simulink model "Grua_MC_R2_FFLimitado_06102026"  (R2025b)
settings: Solver=ode23t  StartTime=0.0  StopTime=628  MaxStep=T_s  RelTol=1e-4
InitFcn:
  | addpath(fileparts(get_param('Grua_MC_R2_FFLimitado_06102026','FileName')),'-begin');
  | run(fullfile(fileparts(get_param('Grua_MC_R2_FFLimitado_06102026','FileName')),'definir_buses_variadores.m'));
  | run(fullfile(fileparts(get_param('Grua_MC_R2_FFLimitado_06102026','FileName')),'parametros_ganancias_cascada_29072026.m'));
  | run(fullfile(fileparts(get_param('Grua_MC_R2_FFLimitado_06102026','FileName')),'configurar_modelo_final_hmi.m'));
  | run(fullfile(fileparts(get_param('Grua_MC_R2_FFLimitado_06102026','FileName')),'configurar_parametros_variadores.m'));
  | 
  | 
  | 
  | 
  | 
  | 
  | 
  | Pvis.Ts_viz=.04;Pvis.enable=true;Pvis.keepFigureOnTerminate=true;Pvis.hmi.captureFolder='D:\AyCD\Chat\Proyecto_grua\Prueba_Completa_MC_20261007\corrida_09';Pvis.hmi.fastDiagnostic=false;Pvis.hmi.testDriver=@operador_dos_traslados_v4;Pvis.hmi.renderPeriod=.20;
StopFcn:
  | guardar_prueba_completa;
undefined symbols (not defined in the file): b_cx, b_cy, b_hb, b_hEb, b_heq, b_t, b_tb, b_teq, b_tw, b_wu, g, H_c, HMI, i_h, i_t, J_heq, J_teq, K_cy, K_tw, k_wu, L_h0, l_hi, M_c_profile, M_s, M_t, MC_FF, nLevels0, omega_hmRATED, r_hd, r_td, slotBlock, T_hbMax, T_hEbMax, T_hmMax, T_s, T_s1, T_tbMax, T_tmMax, tau_hm, tau_tm, traj_duration, traj_x_start, traj_x_target, v_hmaxLoaded, v_hmaxUnloaded, x_tmax, x_tmin, Y_c0, Y_t0, Zbase
libraries: simulink x1, aerolibanimutils x1
(part 4 of 5)

== stateflow chart Grua_MC_R2_FFLimitado_06102026/Automata Supervisor ==
  settings: updateMethod=DISCRETE  sampleTime=T_s1  description=Supervisor autocontenido de grua portacontenedores. Ts1=20 ms. El Nivel 0 de seguridad permanece separado y entrega permisos.
  state REFERENCIAS_CARRO_COMUN [parallel]
    entry:
    [xRef,vxRef,axRef,swayTransferVelocity]=referencias_carro_comunes(xRef,vxRef,axRef,modeCode,manualTrolleyRef,xTrolley,enableTrolleyReg,safetyPermitTrolley,swayControlEnable,lastSwayVelocity,TsSupervisor);
    du:
    [xRef,vxRef,axRef,swayTransferVelocity]=referencias_carro_comunes(xRef,vxRef,axRef,modeCode,manualTrolleyRef,xTrolley,enableTrolleyReg,safetyPermitTrolley,swayControlEnable,lastSwayVelocity,TsSupervisor);
    settings: executionOrder=4
  state OPERACION [parallel]
    settings: executionOrder=3
    state APAGADO
      entry:
      modeCode=0; enableTrolleyReg=false; enableHoistReg=false;
      emergencyBrakeHoistOpenCmd=false; swayControlEnable=false;
      xRef=xTrolley; vxRef=0.0; axRef=0.0;
      yRef=yHoist; vyRef=0.0; ayRef=0.0;
    state LISTO
      entry:
      modeCode=2; enableTrolleyReg=true; enableHoistReg=true;
      xRef=xTrolley; vxRef=0.0; axRef=0.0;
      yRef=yHoist; vyRef=0.0; ayRef=0.0;
    state ARRANQUE
      entry:
      modeCode=1; enableTrolleyReg=false; enableHoistReg=false;
      emergencyBrakeHoistOpenCmd=true;
      xRef=xTrolley; vxRef=0.0; axRef=0.0;
      yRef=yHoist; vyRef=0.0; ayRef=0.0;
    state PREPARAR_ESCANEO_LIDAR
      entry:
      swayControlEnable=false;
      modeCode=9; scanActive=true; profileScanComplete=false; profileValid=false;
      scannedObstacleProfile=-20.0*ones(33,1); scanSampleCounts=zeros(33,1);
      scannedObstacleProfile(33)=0.0; scanSampleCounts(33)=1.0;
      autoCycleComplete=false;
      du:
      enableTrolleyReg=safetyPermitTrolley; enableHoistReg=safetyPermitHoist;
      swayControlEnable=false;
      xRef=xTrolley; vxRef=0.0; axRef=0.0;
      yRef=yHoist; vyRef=min(0.5,0.5*max(0.0,39.7-yHoist)); ayRef=0.0;
      exit: scanActive=false;
    state APROXIMACION_FINAL_MANUAL
      entry: modeCode=3;
      du:
      enableTrolleyReg=safetyPermitTrolley; enableHoistReg=safetyPermitHoist;
      swayControlEnable=swayControlSelect;
      [xRef,vxRef,axRef,yRef,vyRef,ayRef]=referenciaDescensoFinal(autoTargetXLatched,yHoist,vHoist,manualHoistRef,TsSupervisor);
    state MANUAL_SUPERVISADO
      entry: modeCode=3;
      du:
      enableTrolleyReg=safetyPermitTrolley; enableHoistReg=safetyPermitHoist;
      swayControlEnable=swayControlSelect;
      [xRef,vxRef,axRef,yRef,vyRef,ayRef]=referenciasManual(xTrolley,vTrolley,yHoist,vHoist,manualTrolleyRef,manualHoistRef,TsSupervisor);
    state IR_EXTREMO_DERECHO
      entry:
      swayControlEnable=false; modeCode=9; scanActive=true;
      du:
      enableTrolleyReg=safetyPermitTrolley; enableHoistReg=safetyPermitHoist;
      swayControlEnable=false;
      xRef=xTrolley; vxRef=calcularVelocidadBarrido(xTrolley,vTrolley,scanSpeed,true); axRef=0.0;
      yRef=yHoist; vyRef=0.0; ayRef=0.0;
      exit: scanActive=false;
    state BUMPLESS_A_MANUAL
      entry: modeCode=7;
      du:
      enableTrolleyReg=safetyPermitTrolley; enableHoistReg=safetyPermitHoist;
      [xRef,vxRef,axRef,yRef,vyRef,ayRef]=referenciasBumpless(xTrolley,vTrolley,yHoist,vHoist,manualTrolleyRef,manualHoistRef,TsSupervisor);
    state BUMPLESS_A_AUTO
      entry: modeCode=8;
      du:
      enableTrolleyReg=safetyPermitTrolley; enableHoistReg=safetyPermitHoist;
      swayControlEnable=swayControlSelect;
      xRef=xTrolley; vxRef=vTrolley; axRef=aTrolley;
      yRef=yHoist; vyRef=vHoist; ayRef=aHoist;
    state BARRIDO_LIDAR_IZQUIERDA
      entry:
      swayControlEnable=false; modeCode=9; scanActive=true;
      du:
      enableTrolleyReg=safetyPermitTrolley; enableHoistReg=safetyPermitHoist;
      swayControlEnable=false;
      [scannedObstacleProfile,scanSampleCounts]=registrarMuestraLidar(scannedObstacleProfile,scanSampleCounts,lidarX,lidarY);
      xRef=xTrolley; vxRef=calcularVelocidadBarrido(xTrolley,vTrolley,scanSpeed,false); axRef=0.0;
      yRef=yHoist; vyRef=0.0; ayRef=0.0;
      exit: scanActive=false;
    state AUTOMATICO
      entry:
      autoTargetXLatched=autoTargetX;
      autoTargetSurfaceLatched=calcularSuperficieObjetivo(safetyEnvelopeProfile,autoTargetXLatched);
      autoApproachTargetY=calcularObjetivoSeguro(safetyEnvelopeProfile,autoTargetXLatched,loadedState,totalSuspendedMass);
      automaticTargetY=autoApproachTargetY;
      state PLANIFICAR
        entry:
        modeCode=4;
        enableTrolleyReg=safetyPermitTrolley;
        enableHoistReg=safetyPermitHoist;
        swayControlEnable=swayControlSelect;
        [xRef,vxRef,axRef,yRef,vyRef,ayRef]=craneTrajectoryGenerator(true,true,xTrolley,vTrolley,aTrolley,yHoist,vHoist,aHoist,autoTargetXLatched,autoApproachTargetY,safetyEnvelopeProfile,totalSuspendedMass,loadedState,spreaderSwayAngle,spreaderSwayRate,TsSupervisor);
        [vyRef,ayRef]=cerrarLazoPosicionIzaje(yRef,vyRef,ayRef,yHoist,vHoist,loadedState,totalSuspendedMass);
      state EJECUTAR
        du:
        enableTrolleyReg=safetyPermitTrolley;
        enableHoistReg=safetyPermitHoist;
        [xRef,vxRef,axRef,yRef,vyRef,ayRef]=craneTrajectoryGenerator(true,false,xTrolley,vTrolley,aTrolley,yHoist,vHoist,aHoist,autoTargetXLatched,autoApproachTargetY,safetyEnvelopeProfile,totalSuspendedMass,loadedState,spreaderSwayAngle,spreaderSwayRate,TsSupervisor);
        % Por encima de la linea de seguridad se prioriza produccion.
        % Al detener el carro se reactiva antisway antes de autorizar el descenso.
        swayControlEnable=swayControlSelect;
        [vyRef,ayRef]=cerrarLazoPosicionIzaje(yRef,vyRef,ayRef,yHoist,vHoist,loadedState,totalSuspendedMass);
        if abs(xTrolley-autoTargetXLatched)<0.08 && abs(yHoist-autoApproachTargetY)<0.15
        autoCycleComplete=true;
        end
      state MANTENER_OBJETIVO
        entry:
        autoCycleComplete=true;
        du:
        swayControlEnable=swayControlSelect;
        xRef=autoTargetXLatched;
        vxRef=0.0;
        axRef=0.0;
        yRef=autoApproachTargetY;
        vyRef=0.0;
        ayRef=0.0;
      (default) -> PLANIFICAR
      PLANIFICAR -> EJECUTAR : [after(1,tick)]
      EJECUTAR -> MANTENER_OBJETIVO : [abs(xTrolley-autoTargetXLatched)<0.08 && abs(yHoist-autoApproachTargetY)<0.15]
    state FINALIZAR_ESCANEO_LIDAR
      entry:
      swayControlEnable=false;
      modeCode=9; scanActive=false; profileScanComplete=true;
      profileValid=verificarCoberturaPerfil(scanSampleCounts);
      profileMaxY=max(scannedObstacleProfile);
      du:
      swayControlEnable=false;
      enableTrolleyReg=safetyPermitTrolley; enableHoistReg=safetyPermitHoist;
      xRef=xTrolley; vxRef=0.0; axRef=0.0;
      yRef=yHoist; vyRef=0.0; ayRef=0.0;
    state PARADA_NORMAL
      entry: modeCode=5; swayControlEnable=false;
      du:
      enableTrolleyReg=safetyPermitTrolley; enableHoistReg=safetyPermitHoist;
      [xRef,vxRef,axRef,yRef,vyRef,ayRef]=referenciasBumpless(xTrolley,vTrolley,yHoist,vHoist,0.0,0.0,TsSupervisor);
    state RETENCION_FALLA
      entry:
      modeCode=6; enableTrolleyReg=false; enableHoistReg=false;
      swayControlEnable=false;
      xRef=xTrolley; vxRef=0.0; axRef=0.0;
      yRef=yHoist; vyRef=0.0; ayRef=0.0;
    (default) -> APAGADO
    ARRANQUE -> PARADA_NORMAL [order 2] : [cmdStop || ~safetyPermitGlobal]
    LISTO -> PARADA_NORMAL [order 3] : [cmdStop || ~safetyPermitGlobal]
    RETENCION_FALLA -> APAGADO : [cmdReset && safetyPermitGlobal && ~trackingFault && ~loadSequenceFault]
    PARADA_NORMAL -> APAGADO : [allStopped]
    APAGADO -> ARRANQUE : [cmdStart && safetyPermitGlobal && configValid]
    ARRANQUE -> LISTO [order 1] : [safetyPermitTrolley && safetyPermitHoist && after(5,tick)]
    FINALIZAR_ESCANEO_LIDAR -> LISTO [order 1] : [allStopped]
    LISTO -> MANUAL_SUPERVISADO [order 1] : [~modeAutoReq && (~scanProfileReq || profileScanComplete)]
    LISTO -> RETENCION_FALLA [order 4] : [trackingFault || loadSequenceFault]
    MANUAL_SUPERVISADO -> PREPARAR_ESCANEO_LIDAR [order 4] : [scanProfileReq && ~profileScanComplete && ~loadedState && allStopped]
    LISTO -> AUTOMATICO [order 2] : [modeAutoReq && cmdAutoStart && profileValid && autoEntryHeightOK && ~overloadDetected]
    LISTO -> PREPARAR_ESCANEO_LIDAR [order 5] : [scanProfileReq && ~profileScanComplete && ~loadedState]
    ARRANQUE -> RETENCION_FALLA [order 3] : [trackingFault || loadSequenceFault]
    BUMPLESS_A_MANUAL -> MANUAL_SUPERVISADO [order 1] : [abs(vTrolley)<0.10 && abs(vHoist)<0.03 && ~autoCycleComplete]
    APROXIMACION_FINAL_MANUAL -> MANUAL_SUPERVISADO [order 1] : [~loadedState]
    PREPARAR_ESCANEO_LIDAR -> PARADA_NORMAL [order 2] : [cmdStop || ~safetyPermitGlobal]
    PREPARAR_ESCANEO_LIDAR -> RETENCION_FALLA [order 3] : [loadSequenceFault]
    MANUAL_SUPERVISADO -> PARADA_NORMAL [order 2] : [cmdStop || ~safetyPermitGlobal]
    PREPARAR_ESCANEO_LIDAR -> IR_EXTREMO_DERECHO [order 1] : [yHoist>=39.65 && abs(vHoist)<0.05]
    BUMPLESS_A_MANUAL -> APROXIMACION_FINAL_MANUAL [order 4] : [abs(vTrolley)<0.10 && abs(vHoist)<0.03 && autoCycleComplete]
    APROXIMACION_FINAL_MANUAL -> PARADA_NORMAL [order 2] : [cmdStop || ~safetyPermitGlobal]
    APROXIMACION_FINAL_MANUAL -> RETENCION_FALLA [order 3] : [trackingFault || loadSequenceFault]
    IR_EXTREMO_DERECHO -> PARADA_NORMAL [order 2] : [cmdStop || ~safetyPermitGlobal]
    IR_EXTREMO_DERECHO -> RETENCION_FALLA [order 3] : [loadSequenceFault]
    IR_EXTREMO_DERECHO -> BARRIDO_LIDAR_IZQUIERDA [order 1] : [normalLimitXMax || (xTrolley>=48.40 && abs(vTrolley)<0.15)]
    MANUAL_SUPERVISADO -> RETENCION_FALLA [order 3] : [trackingFault || loadSequenceFault]
    BUMPLESS_A_MANUAL -> PARADA_NORMAL [order 2] : [cmdStop || ~safetyPermitGlobal]
    MANUAL_SUPERVISADO -> BUMPLESS_A_AUTO [order 1] : [modeAutoReq && cmdAutoStart && ~overloadDetected && profileValid && autoEntryHeightOK && ~operatorOverride && ~autoCycleComplete]
    BUMPLESS_A_AUTO -> PARADA_NORMAL [order 2] : [cmdStop || ~safetyPermitGlobal]
    BUMPLESS_A_AUTO -> RETENCION_FALLA [order 3] : [trackingFault || loadSequenceFault]
    BUMPLESS_A_MANUAL -> RETENCION_FALLA [order 3] : [trackingFault || loadSequenceFault]
    AUTOMATICO -> BUMPLESS_A_MANUAL [order 1] : [operatorOverride || ~modeAutoReq || autoCycleComplete]
    BARRIDO_LIDAR_IZQUIERDA -> PARADA_NORMAL [order 2] : [cmdStop || ~safetyPermitGlobal]
    BARRIDO_LIDAR_IZQUIERDA -> RETENCION_FALLA [order 3] : [loadSequenceFault]
    BARRIDO_LIDAR_IZQUIERDA -> FINALIZAR_ESCANEO_LIDAR [order 1] : [normalLimitXMin || (xTrolley<=-24.50 && abs(vTrolley)<0.15)]
    BUMPLESS_A_AUTO -> AUTOMATICO [order 1] : [after(2,tick)]
    FINALIZAR_ESCANEO_LIDAR -> PARADA_NORMAL [order 2] : [cmdStop || ~safetyPermitGlobal]
    FINALIZAR_ESCANEO_LIDAR -> RETENCION_FALLA [order 3] : [loadSequenceFault]
    AUTOMATICO -> PARADA_NORMAL [order 2] : [cmdStop || ~safetyPermitGlobal]
    AUTOMATICO -> RETENCION_FALLA [order 3] : [trackingFault || loadSequenceFault]
  state FRENOS [parallel]
    settings: executionOrder=5
    state FRENO_IZAJE [parallel]
      settings: executionOrder=2
      state HB_APLICADO
        entry: brakeHoistOpenCmd=false;
      state HB_PRUEBA_TORQUE
        entry: brakeHoistOpenCmd=false;
      state HB_ABIERTO
        entry: brakeHoistOpenCmd=true;
      state HB_APLICANDO
        entry: brakeHoistOpenCmd=true;
        du: brakeHoistOpenCmd=safetyPermitHoist && (abs(vHoist)>=0.03 || abs(yRef-yHoist)>0.05);
      (default) -> HB_APLICADO
      HB_APLICADO -> HB_PRUEBA_TORQUE : [enableHoistReg && (abs(vyRef)>0.01 || abs(yRef-yHoist)>0.05) && safetyPermitHoist]
      HB_APLICANDO -> HB_APLICADO : [abs(vHoist)<0.03 && abs(yRef-yHoist)<=0.05]
      HB_PRUEBA_TORQUE -> HB_APLICADO [order 2] : [after(50,tick)]
      HB_PRUEBA_TORQUE -> HB_ABIERTO [order 1] : [torqueProvenHoist]
      HB_ABIERTO -> HB_APLICANDO : [~enableHoistReg || (modeCode~=4 && abs(vyRef)<=0.01 && abs(yRef-yHoist)<=0.05) || ~safetyPermitHoist]
    state FRENO_CARRO [parallel]
      settings: executionOrder=1
      state TB_APLICADO
        entry: brakeTrolleyOpenCmd=false;
      state TB_PRUEBA_TORQUE
        entry: brakeTrolleyOpenCmd=false;
      state TB_ABIERTO
        entry: brakeTrolleyOpenCmd=true;
      state TB_APLICANDO
        entry: brakeTrolleyOpenCmd=true;
        du: brakeTrolleyOpenCmd=safetyPermitTrolley && (abs(vTrolley)>=0.03 || abs(xRef-xTrolley)>0.03);
      (default) -> TB_APLICADO
      TB_APLICANDO -> TB_APLICADO : [abs(vTrolley)<0.03 && abs(xRef-xTrolley)<=0.03]
      TB_PRUEBA_TORQUE -> TB_APLICADO [order 2] : [after(50,tick)]
      TB_APLICADO -> TB_PRUEBA_TORQUE : [enableTrolleyReg && (abs(vxRef)>0.01 || abs(xRef-xTrolley)>0.03) && safetyPermitTrolley]
      TB_PRUEBA_TORQUE -> TB_ABIERTO [order 1] : [torqueProvenTrolley]
      TB_ABIERTO -> TB_APLICANDO : [~enableTrolleyReg || (abs(vxRef)<=0.01 && abs(xRef-xTrolley)<=0.03) || ~safetyPermitTrolley]
  state INTERLOCKS [parallel]
    du:
    [cmdTwistlockClose,cmdTwistlockOpen,vTrolley,aTrolley,aHoist,normalLimitYMin,normalLimitYMax,trackingFault,torqueProvenTrolley,torqueProvenHoist]=procesarEntradasCrudas(twistlockButton,omegaTrolley,vHoist,yHoist,torqueTrolleyRaw,torqueHoistRaw,xTrolley,xRef,yRef,modeCode,TsSupervisor);
    scanProfileReq=retenerSolicitudHMI(hmiScanRequestRaw,scanActive,profileScanComplete,cmdStop,cmdReset);
    ropeSlack=detectarCuerdaFloja(ropeTension);
    if profileValid && ~scanActive && loadedState~=previousLoadedState
    scannedObstacleProfile=actualizarPerfilPorCarga(scannedObstacleProfile,xTrolley,loadedState);
    end
    previousLoadedState=loadedState;
    safetyEnvelopeProfile=calcularEnvolventeLocal(scannedObstacleProfile);
    autoEntryHeightOK=profileValid && yHoist>=calcularObjetivoSeguro(safetyEnvelopeProfile,xTrolley,loadedState,totalSuspendedMass);
    autoTargetSurfaceLatched=calcularSuperficieObjetivo(safetyEnvelopeProfile,autoTargetXLatched);
    autoApproachTargetY=calcularObjetivoSeguro(safetyEnvelopeProfile,autoTargetXLatched,loadedState,totalSuspendedMass);
    automaticTargetY=autoApproachTargetY;
    if ~modeAutoReq
    autoCycleComplete=false;
    end
    if ~scanProfileReq && ~scanActive
    profileScanComplete=false;
    end
    [loadSupported,operatorOverride,allStopped,atAutoTargetX,atAutoTargetY]=calcularFlagsSupervisor(ropeTension,twistlocksClosedFb,joyTrolley,joyHoist,xTrolley,vTrolley,yHoist,vHoist,autoTargetXLatched,autoApproachTargetY);
    allStopped=allStopped && abs(vxRef)<0.01 && abs(axRef)<0.03 && abs(xRef-xTrolley)<0.08 && abs(swayTransferVelocity)<0.01;
    [manualTrolleyRef,manualHoistRef,vHoistMax]=calcularMandoManual(joyTrolley,joyHoist,loadedState,overloadDetected,totalSuspendedMass,normalLimitXMin,normalLimitXMax,normalLimitYMin,normalLimitYMax);
    profileMaxY=max(scannedObstacleProfile);
    clearanceLineY=max(manualToAutoHeight,min(40.0,profileMaxY+5.18));
    clearanceOK=calcularDespeje(yHoist,clearanceLineY,totalSuspendedMass);
    [alarmCodeCalc,faultCodeCalc]=calcularCodigos(overloadDetected,trackingFault,loadSequenceFault,safetyPermitGlobal);
    watchdogToggle=~watchdogToggle;
    [spreaderStable,spreaderStableCounter]=evaluarEstabilidadSpreader(spreaderSwayAngle,spreaderSwayRate,contact4,cmdTwistlockClose,spreaderStableCounter,TsSupervisor);
    [postLockStable,postLockStableCounter]=evaluarEstabilidadSpreader(spreaderSwayAngle,spreaderSwayRate,contact4,twistlocksClosedFb,postLockStableCounter,TsSupervisor);
    [manualTrolleyRef,manualHoistRef]=aplicarRetencionToma(manualTrolleyRef,manualHoistRef,twistlocksClosedFb,contact4,postLockStable);
    settings: executionOrder=1
  state CARGA_Y_TWISTLOCKS [parallel]
    settings: executionOrder=2
    state VACIO
      entry:
      loadedState=false; overloadDetected=false; pickupModeActive=false;
      twistlockCloseCmd=false; twistlockOpenCmd=false;
      massEstimationEnable=false; massEstimateValid=false;
      estimatedContainerMass=0.0; totalSuspendedMass=15000.0;
    state CERRANDO_TWISTLOCKS
      entry: twistlockCloseCmd=true; twistlockOpenCmd=false;
      exit: twistlockCloseCmd=false;
    state ESPERAR_ESTABILIZACION_SPREADER
      entry:
      twistlockCloseCmd=false; twistlockOpenCmd=false;
      du:
      twistlockCloseCmd=false; twistlockOpenCmd=false;
    state DESPEGUE_SUAVE
      entry:
      loadedState=true; pickupModeActive=true; massEstimationEnable=false;
    state PESAJE
      entry:
      massEstimationEnable=true; pickupModeActive=true;
      massAccum=0.0; massSampleCount=0.0;
      du:
      massAccum=massAccum+Estimar_Masa(ropeTension,twistlocksClosedFb);
      massSampleCount=massSampleCount+1.0;
      estimatedContainerMass=massAccum/max(1.0,massSampleCount);
      totalSuspendedMass=15000.0+estimatedContainerMass;
      exit: massEstimationEnable=false; pickupModeActive=false;
    state CARGADO
      entry:
      loadedState=true; overloadDetected=false; pickupModeActive=false;
      massEstimateValid=true;
    state SOBRECARGA
      entry:
      loadedState=true; overloadDetected=true; pickupModeActive=false;
      massEstimateValid=true;
    state ABRIENDO_TWISTLOCKS
      entry: twistlockOpenCmd=true; twistlockCloseCmd=false;
      exit: twistlockOpenCmd=false;
    state FALLA_TWISTLOCK
      entry: loadSequenceFault=true; twistlockCloseCmd=false; twistlockOpenCmd=false;
      exit: loadSequenceFault=false;
    ESPERAR_ESTABILIZACION_SPREADER -> CERRANDO_TWISTLOCKS [order 1] : [spreaderStable && cmdTwistlockClose && contact4 && safetyPermitHoist]
    (default) -> VACIO
    ESPERAR_ESTABILIZACION_SPREADER -> VACIO [order 2] : [~cmdTwistlockClose || ~contact4]
    VACIO -> ESPERAR_ESTABILIZACION_SPREADER : [cmdTwistlockClose && contact4 && safetyPermitHoist]
    ABRIENDO_TWISTLOCKS -> VACIO [order 1] : [~twistlocksClosedFb]
    FALLA_TWISTLOCK -> VACIO : [cmdReset && ~twistlocksClosedFb]
    CERRANDO_TWISTLOCKS -> FALLA_TWISTLOCK [order 2] : [after(100,tick)]
    CERRANDO_TWISTLOCKS -> DESPEGUE_SUAVE [order 1] : [twistlocksClosedFb]
    ESPERAR_ESTABILIZACION_SPREADER -> FALLA_TWISTLOCK [order 3] : [~safetyPermitHoist || trackingFault]
    DESPEGUE_SUAVE -> ABRIENDO_TWISTLOCKS [order 2] : [cmdTwistlockOpen && contact4]
    DESPEGUE_SUAVE -> PESAJE [order 1] : [~ropeSlack && abs(vHoist)<0.20 && abs(aHoist)<0.05]
    PESAJE -> CARGADO [order 2] : [after(25,tick) && estimatedContainerMass<=50000.0]
    PESAJE -> SOBRECARGA [order 1] : [after(25,tick) && estimatedContainerMass>50000.0]
    SOBRECARGA -> ABRIENDO_TWISTLOCKS : [cmdTwistlockOpen && contact4]
    CARGADO -> ABRIENDO_TWISTLOCKS : [cmdTwistlockOpen && contact4]
    ABRIENDO_TWISTLOCKS -> FALLA_TWISTLOCK [order 2] : [after(100,tick)]
  state DIAGNOSTICO [parallel]
    settings: executionOrder=6
    state DIAG_OK
      du: alarmCode=0.0; faultCode=0.0;
    state ALARMA
      du: alarmCode=alarmCodeCalc; faultCode=0.0;
    state FALLA
      du: faultCode=faultCodeCalc;
    (default) -> DIAG_OK
    DIAG_OK -> ALARMA [order 1] : [overloadDetected]
    FALLA -> DIAG_OK : [cmdReset && ~trackingFault && ~loadSequenceFault && safetyPermitGlobal]
    DIAG_OK -> FALLA [order 2] : [trackingFault || loadSequenceFault || ~safetyPermitGlobal]
    ALARMA -> DIAG_OK [order 2] : [cmdReset && ~overloadDetected]
    ALARMA -> FALLA [order 1] : [trackingFault || loadSequenceFault || ~safetyPermitGlobal]
  data: yReference function_input; velocityPlan function_input; accelerationPlan function_input; yMeasured function_input; velocityMeasured function_input; loaded function_input; velocityCommand function_output; accelerationCommand function_output; totalMassKg function_input; angle function_input; rate function_input; contact function_input; closeRequest function_input; counter function_input; Ts function_input; stable function_output; counter function_output; vxCmd function_input; vyCmd function_input; twistClosed function_input; contact function_input; stable function_input; vxSafe function_output; vySafe function_output; profile function_input; xTarget function_input; surfaceY function_output; buttonRaw function_input; omegaT function_input; vH function_input; yH function_input; torqueTRaw function_input; torqueHRaw function_input; x function_input; xReference function_input; yReference function_input; currentMode function_input; Ts function_input; closeRequest function_output; openRequest function_output; vT function_output; aT function_output; aH function_output; yMin function_output; yMax function_output; trackFault function_output; torqueTProven function_output; torqueHProven function_output; profileIn function_input; countIn function_input; xSensor function_input; ySensor function_input; profileOut function_output; countOut function_output; sampleCounts function_input; valid function_output; x function_input; v function_input; speedRequest function_input; toRight function_input; velocityCommand function_output; profile function_input; envelope function_output; profileIn function_input; x function_input; loadedNow function_input; profileOut function_output; envelope function_input; xTarget function_input; loaded function_input; massKg function_input; yGoal function_output; raw function_input; active function_input; complete function_input; stop function_input; reset function_input; request function_output; ropeTension function_input; ropeSlack function_output; ropeTension function_input; twistlocksClosed function_input; joyX function_input; joyY function_input; x function_input; vx function_input; y function_input; vy function_input; xTarget function_input; yTarget function_input; loadSupported function_output; operatorOverride function_output; allStopped function_output; atTargetX function_output; atTargetY function_output; joyX function_input; joyY function_input; loaded function_input; overload function_input; totalMass function_input; xMinLimit function_input; xMaxLimit function_input; yMinLimit function_input; yMaxLimit function_input; vxManual function_output; vyManual function_output; vyMax function_output; y function_input; clearanceLine function_input; totalMass function_input; clearanceOK function_output; overload function_input; trackingFault function_input; loadFault function_input; safetyGlobal function_input; alarmCode function_output; faultCode function_output; xPlan function_input; vPlan function_input; aPlan function_input; mode function_input; manualVelocity function_input; xMeasured function_input; enabled function_input; permit function_input; E function_input; lastSw function_input; Ts function_input; xr function_output; vr function_output; ar function_output; transfer function_output; enable function_input; reset function_input; xPos function_input; xVel function_input; xAcc function_input; yPos function_input; yVel function_input; yAcc function_input; xTarget function_input; yTarget function_input; obstacleProfile function_input; suspendedMassKg function_input; loaded function_input; swayAngle function_input; swayRate function_input; Ts function_input; xRef function_output; vxRef function_output; axRef function_output; yRef function_output; vyRef function_output; ayRef function_output; x function_input; vx function_input; y function_input; vy function_input; vxCmd function_input; vyCmd function_input; Ts function_input; xRef function_output; vxRef function_output; axRef function_output; yRef function_output; vyRef function_output; ayRef function_output; x function_input; vx function_input; y function_input; vy function_input; vxTarget function_input; vyTarget function_input; Ts function_input; xRef function_output; vxRef function_output; axRef function_output; yRef function_output; vyRef function_output; ayRef function_output; xTarget function_input; y function_input; vy function_input; vyCmd function_input; Ts function_input; xRef function_output; vxRef function_output; axRef function_output; yRef function_output; vyRef function_output; ayRef function_output; F_hw function_input; TLK_Close_FB function_input; masa function_output; cmdStart input boolean size=1; cmdStop input boolean size=1; modeAutoReq input boolean size=1; cmdAutoStart input boolean size=1; cmdReset input boolean size=1; swayControlSelect input boolean size=1; configValid input boolean size=1; twistlockButton input double; contact4 input boolean size=1; twistlocksClosedFb input boolean size=1; normalLimitXMin input boolean size=1; normalLimitXMax input boolean size=1; safetyPermitGlobal input boolean size=1; safetyPermitTrolley input boolean size=1; safetyPermitHoist input boolean size=1; joyTrolley input double size=1; joyHoist input double size=1; xTrolley input double size=1; omegaTrolley input double; yHoist input double size=1; vHoist input double size=1; ropeTension input double size=1; torqueTrolleyRaw input double; torqueHoistRaw input double; autoTargetX input double size=1; enableTrolleyReg output boolean size=1 =0; enableHoistReg output boolean size=1 =0; brakeTrolleyOpenCmd output boolean size=1 =0; brakeHoistOpenCmd output boolean size=1 =0; emergencyBrakeHoistOpenCmd output boolean size=1 =0; twistlockCloseCmd output boolean size=1 =0; twistlockOpenCmd output boolean size=1 =0; swayControlEnable output boolean size=1 =0; loadedState output boolean size=1 =0; overloadDetected output boolean size=1 =0; watchdogToggle output boolean size=1 =0; xRef output double size=1 =0; vxRef output double size=1 =0; axRef output double size=1 =0; yRef output double size=1 =0; vyRef output double size=1 =0; ayRef output double size=1 =0; modeCode output double size=1 =0; alarmCode output double size=1 =0; faultCode output double size=1 =0; ropeSlack local boolean size=1 =0; loadSupported local boolean size=1 =0; operatorOverride local boolean size=1 =0; allStopped local boolean size=1 =0; atAutoTargetX local boolean size=1 =0; atAutoTargetY local boolean size=1 =0; clearanceOK local boolean size=1 =0; loadSequenceFault local boolean size=1 =0; massEstimationEnable local boolean size=1 =0; pickupModeActive local boolean size=1 =0; vHoistMax local double size=1 =0; totalSuspendedMass local double size=1 =15000; alarmCodeCalc local double size=1 =0; faultCodeCalc local double size=1 =0; TsSupervisor local double size=1 =0.02; manualToAutoHeight input double size=1; finalApproachDistance input double size=1; autoApproachTargetY local double size=1 =0; autoCycleComplete local boolean size=1 =0; spreaderSwayAngle input double size=1; spreaderSwayRate input double size=1; hmiScanRequestRaw input boolean; spreaderStable local boolean size=1 =0; spreaderStableCounter local double size=1 =0; postLockStable local boolean size=1 =0; postLockStableCounter local double size=1 =0; cmdTwistlockClose local boolean size=1 =false; cmdTwistlockOpen local boolean size=1 =false; vTrolley local double size=1 =0.0; aTrolley output double size=1 =0.0; aHoist output double size=1 =0.0; trackingFault output boolean size=1 =false; torqueProvenTrolley output boolean size=1 =false; torqueProvenHoist output boolean size=1 =false; autoTargetXLatched local double =0.0; massAccum local double =0.0; massSampleCount local double =0.0; autoTargetSurfaceLatched local double =0.0; lidarX input double size=1; lidarY input double size=1; scanSpeed input double size=1; profileScanComplete output boolean =false; profileValid output boolean =false; scanActive output boolean =false; scannedObstacleProfile output double size=[33 1] =-20.0*ones(33,1); profileMaxY output double =-20.0; automaticTargetY output double =-20.0; scanSampleCounts local double size=[33 1] =zeros(33,1); clearanceLineY output double =0.0; estimatedContainerMass output double size=1 =0; massEstimateValid output boolean size=1 =0; normalLimitYMin output boolean size=1 =false; normalLimitYMax output boolean size=1 =false; manualTrolleyRef output double size=1 =0; manualHoistRef output double size=1 =0; scanProfileReq local boolean size=1; safetyEnvelopeProfile output double size=[33 1] =zeros(33,1); previousLoadedState local boolean size=1 =false; autoEntryHeightOK local boolean size=1 =false; lastSwayVelocity input; swayTransferVelocity output =0
  function [velocityCommand,accelerationCommand] = cerrarLazoPosicionIzaje(yReference,velocityPlan,accelerationPlan,yMeasured,velocityMeasured,loaded,totalMassKg):
    | function [velocityCommand,accelerationCommand] = cerrarLazoPosicionIzaje(yReference,velocityPlan,accelerationPlan,yMeasured,velocityMeasured,loaded,totalMassKg)
    | %#codegen
    | positionGain=0.60;
    | if loaded
    |     massUse=min(65000.0,max(15000.0,totalMassKg));
    |     velocityLimit=min(3.0,max(1.5,97500.0/massUse)); correctionLimit=0.20;
    | else
    |     velocityLimit=3.00; correctionLimit=1.50;
    | end
    | positionError=yReference-yMeasured;
    | if abs(positionError)<=0.05
    |     positionCorrection=0.0;
    | else
    |     effectiveError=positionError-sign(positionError)*0.05;
    |     positionCorrection=min(correctionLimit,max(-correctionLimit,positionGain*effectiveError));
    | end
    | velocityCommand=min(velocityLimit,max(-velocityLimit,velocityPlan+positionCorrection));
    | accelerationCommand=min(0.25,max(-0.25,accelerationPlan+0.05*(velocityCommand-velocityMeasured)));
    | end
  function [stable,counter]=evaluarEstabilidadSpreader(angle,rate,contact,closeRequest,counter,Ts):
    | function [stable,counter]=evaluarEstabilidadSpreader(angle,rate,contact,closeRequest,counter,Ts)
    | %#codegen
    | % Tolerancias: 0.57 grados y 1.15 grados/s durante 1 segundo.
    | % Se limita la oscilacion, no una pequena inclinacion estacionaria.
    | angleLimit=0.010; rateLimit=0.020;
    | requiredSamples=max(1.0,ceil(1.0/max(0.001,Ts)));
    | insideLimits=contact && closeRequest && abs(angle)<=angleLimit && abs(rate)<=rateLimit;
    | if insideLimits
    |     counter=min(requiredSamples,counter+1.0);
    | else
    |     counter=0.0;
    | end
    | stable=counter>=requiredSamples;
    | end
  function [vxSafe,vySafe]=aplicarRetencionToma(vxCmd,vyCmd,twistClosed,contact,stable):
    | function [vxSafe,vySafe]=aplicarRetencionToma(vxCmd,vyCmd,twistClosed,contact,stable)
    | %#codegen
    | holdPickup=twistClosed && contact && ~stable;
    | if holdPickup
    |     vxSafe=0.0; vySafe=0.0;
    | else
    |     vxSafe=vxCmd; vySafe=vyCmd;
    | end
    | end
  function surfaceY = calcularSuperficieObjetivo(profile,xTarget):
    | function surfaceY = calcularSuperficieObjetivo(profile,xTarget)
    | %#codegen
    | xMin=-30.0; slotWidth=2.44; halfContainerWidth=1.22; overlapTolerance=1.0e-6;
    | loadMin=xTarget-halfContainerWidth;
    | loadMax=xTarget+halfContainerWidth;
    | surfaceY=-20.0;
    | for k=1:33
    |     slotMin=xMin+double(k-1)*slotWidth;
    |     slotMax=slotMin+slotWidth;
    |     if slotMax>loadMin+overlapTolerance && slotMin<loadMax-overlapTolerance
    |         surfaceY=max(surfaceY,profile(k));
    |     end
    | end
    | end
  function [closeRequest,openRequest,vT,aT,aH,yMin,yMax,trackFault,torqueTProven,torqueHProven] = procesarEntradasCrudas(buttonRaw,omegaT,vH,yH,torqueTRaw,torqueHRaw,x,xReference,yReference,currentMode,Ts):
    | function [closeRequest,openRequest,vT,aT,aH,yMin,yMax,trackFault,torqueTProven,torqueHProven] = procesarEntradasCrudas(buttonRaw,omegaT,vH,yH,torqueTRaw,torqueHRaw,x,xReference,yReference,currentMode,Ts)
    | %#codegen
    | persistent initialized previousButton toggleState previousVT previousVH trackingTimer
    | if isempty(initialized)
    |     initialized=true; previousButton=false; toggleState=false;
    |     previousVT=0.0; previousVH=0.0;
    |     trackingTimer=0.0;
    | end
    | sampleTime=max(0.001,Ts);
    | button=buttonRaw>=0.5;
    | if button && ~previousButton
    |     toggleState=~toggleState;
    | end
    | previousButton=button; closeRequest=toggleState; openRequest=~toggleState;
    | vT=0.5*omegaT;
    | aT=min(10.0,max(-10.0,(vT-previousVT)/sampleTime));
    | aH=min(10.0,max(-10.0,(vH-previousVH)/sampleTime));
    | previousVT=vT; previousVH=vH;
    | yMin=yH<=-20.0; yMax=yH>=40.0;
    | torqueTProven=abs(torqueTRaw)>=20.0;
    | torqueHProven=abs(torqueHRaw)>=100.0;
    | badX=abs(xReference-x)>2.5;
    | badY=abs(yReference-yH)>max(1.00,2.0*abs(vH)+0.25);
    | automaticMode=currentMode==4.0 || currentMode==8.0;
    | if automaticMode && (badX || badY)
    |     trackingTimer=trackingTimer+sampleTime;
    | else
    |     trackingTimer=0.0;
    | end
    | trackFault=trackingTimer>=3.0;
    | end
  function [profileOut,countOut] = registrarMuestraLidar(profileIn,countIn,xSensor,ySensor):
    | function [profileOut,countOut] = registrarMuestraLidar(profileIn,countIn,xSensor,ySensor)
    | %#codegen
    | profileOut=profileIn; countOut=countIn;
    | xMin=-30.0; slotWidth=2.44;
    | slot=floor((xSensor-xMin)/slotWidth)+1;
    | if slot>=1 && slot<=33
    |     sampleY=min(40.0,max(-20.0,ySensor));
    |     if countOut(slot)<0.5
    |         profileOut(slot)=sampleY;
    |     else
    |         profileOut(slot)=max(profileOut(slot),sampleY);
    |     end
    |     countOut(slot)=countOut(slot)+1.0;
    | end
    | end
  function valid = verificarCoberturaPerfil(sampleCounts):
    | function valid = verificarCoberturaPerfil(sampleCounts)
    | %#codegen
    | valid=true;
    | for k=1:33
    |     if sampleCounts(k)<1.0
    |         valid=false;
    |     end
    | end
    | end
  function velocityCommand = calcularVelocidadBarrido(x,v,speedRequest,toRight):
    | function velocityCommand = calcularVelocidadBarrido(x,v,speedRequest,toRight)
    | speedLimit=min(2.0,max(0.2,abs(speedRequest)));
    | brakingAcceleration=0.15;
    | if toRight
    |     remaining=max(0.0,48.7-x); direction=1.0;
    | else
    |     remaining=max(0.0,x+24.6); direction=-1.0;
    | end
    | velocityCommand=direction*min(speedLimit,sqrt(2.0*brakingAcceleration*remaining));
    | if remaining<=0.0
    |     if toRight && v>0.15
    |         velocityCommand=0.0;
    |     elseif ~toRight && v<-0.15
    |         velocityCommand=0.0;
    |     else
    |         velocityCommand=0.0;
    |     end
    | end
    | end
  function envelope=calcularEnvolventeLocal(profile):
    | function envelope=calcularEnvolventeLocal(profile)
    | %#codegen
    | envelope=zeros(33,1);
    | for k=1:33
    |     left=max(1,k-1); right=min(33,k+1);
    |     envelope(k)=max(profile(left:right));
    | end
    | end
  function profileOut=actualizarPerfilPorCarga(profileIn,x,loadedNow):
    | function profileOut=actualizarPerfilPorCarga(profileIn,x,loadedNow)
    | %#codegen
    | profileOut=profileIn;
    | slot=min(33,max(1,floor((x+30.0)/2.44)+1));
    | if loadedNow
    |     profileOut(slot)=profileOut(slot)-2.59;
    | else
    |     profileOut(slot)=profileOut(slot)+2.59;
    | end
    | end
  function yGoal=calcularObjetivoSeguro(envelope,xTarget,loaded,massKg):
    | function yGoal=calcularObjetivoSeguro(envelope,xTarget,loaded,massKg)
    | %#codegen
    | surface=calcularSuperficieObjetivo(envelope,xTarget);
    | base=surface+2.59+2.59*double(loaded);
    | rope=max(5.0,min(65.0,45.0-base));
    | khw=236.0e6/(2.0*rope+110.0);
    | stretch=max(15000.0,min(65000.0,massKg))*9.80665/(4.0*khw);
    | yGoal=base+stretch;
    | end
  function request=retenerSolicitudHMI(raw,active,complete,stop,reset):
    | function request=retenerSolicitudHMI(raw,active,complete,stop,reset)
    | %#codegen
    | persistent pending previousRaw
    | if isempty(pending), pending=false; previousRaw=false; end
    | if stop || reset || complete
    |  pending=false;
    | elseif raw && ~previousRaw && ~active
    |  pending=true;
    | end
    | previousRaw=raw; request=pending;
    | end
  function ropeSlack = detectarCuerdaFloja(ropeTension):
    | function ropeSlack = detectarCuerdaFloja(ropeTension)
    | %#codegen
    | persistent slackMemory
    | if isempty(slackMemory)
    | slackMemory=true;
    | end
    | if slackMemory
    |     if ropeTension>15000.0
    | slackMemory=false;
    | end
    | else
    |     if ropeTension<12000.0
    | slackMemory=true;
    | end
    | end
    | ropeSlack=slackMemory;
    | end
  function [loadSupported,operatorOverride,allStopped,atTargetX,atTargetY] = calcularFlagsSupervisor(ropeTension,twistlocksClosed,joyX,joyY,x,vx,y,vy,xTarget,yTarget):
    | function [loadSupported,operatorOverride,allStopped,atTargetX,atTargetY] = calcularFlagsSupervisor(ropeTension,twistlocksClosed,joyX,joyY,x,vx,y,vy,xTarget,yTarget)
    | %#codegen
    | loadSupported=twistlocksClosed && ropeTension>30000.0;
    | operatorOverride=abs(joyX)>0.08 || abs(joyY)>0.08;
    | allStopped=abs(vx)<0.03 && abs(vy)<0.03;
    | atTargetX=abs(x-xTarget)<0.03;
    | atTargetY=abs(y-yTarget)<0.10;
    | end
  function [vxManual,vyManual,vyMax] = calcularMandoManual(joyX,joyY,loaded,overload,totalMass,xMinLimit,xMaxLimit,yMinLimit,yMaxLimit):
    | function [vxManual,vyManual,vyMax] = calcularMandoManual(joyX,joyY,loaded,overload,totalMass,xMinLimit,xMaxLimit,yMinLimit,yMaxLimit)
    | %#codegen
    | if loaded
    |     massUse=min(65000.0,max(15000.0,totalMass));
    |     vyMax=min(3.0,max(1.5,97500.0/massUse));
    | else
    |     vyMax=3.0;
    | end
    | if abs(joyX)<=0.05, vxManual=0.0; else, vxManual=4.0*joyX; end
    | if abs(joyY)<=0.05, vyManual=0.0; else, vyManual=vyMax*joyY; end
    | vxManual=min(4.0,max(-4.0,vxManual));
    | vyManual=min(vyMax,max(-vyMax,vyManual));
    | if overload
    |     vxManual=0.0;
    |     vyMax=0.15; % 10%% de la velocidad nominal cargada
    |     vyManual=min(0.0,max(-vyMax,vyManual));
    | end
    | if (xMinLimit && vxManual<0.0) || (xMaxLimit && vxManual>0.0), vxManual=0.0; end
    | if (yMinLimit && vyManual<0.0) || (yMaxLimit && vyManual>0.0), vyManual=0.0; end
    | end
  function clearanceOK = calcularDespeje(y,clearanceLine,totalMass):
    | function clearanceOK = calcularDespeje(y,clearanceLine,totalMass)
    | %#codegen
    | massUse=min(65000.0,max(15000.0,totalMass));
    | lh=max(5.0,min(65.0,45.0-y));
    | khw=236.0e6/(2.0*lh+110.0);
    | cableStretch=massUse*9.80665/(4.0*khw);
    | clearanceOK=(y-cableStretch)>=clearanceLine;
    | end
  function [alarmCode,faultCode] = calcularCodigos(overload,trackingFault,loadFault,safetyGlobal):
    | function [alarmCode,faultCode] = calcularCodigos(overload,trackingFault,loadFault,safetyGlobal)
    | %#codegen
    | alarmCode=0.0;
    | if overload
    |     alarmCode=1.0;
    | end
    | faultCode=0.0;
    | if trackingFault
    |     faultCode=10.0;
    | elseif loadFault
    |     faultCode=11.0;
    | elseif ~safetyGlobal
    |     faultCode=12.0;
    | end
    | end
  function [xr,vr,ar,transfer]=referencias_carro_comunes(xPlan,vPlan,aPlan,mode,manualVelocity,xMeasured,enabled,permit,E,lastSw,Ts):
    | function [xr,vr,ar,transfer]=referencias_carro_comunes(xPlan,vPlan,aPlan,mode,manualVelocity,xMeasured,enabled,permit,E,lastSw,Ts)
    | %#codegen
    | % N1: objetivos distintos; una sola memoria x/v/a, sin predictor de planta.
    | persistent initialized x v a oldE bias
    | if isempty(initialized)
    |  initialized=true;x=xMeasured;v=0.0;a=0.0;oldE=false;bias=0.0;
    | end
    | h=max(0.001,Ts);amax=0.30;jmax=0.50;
    | if ~enabled || ~permit
    |  x=xMeasured;v=0.0;a=0.0;bias=0.0;oldE=false;
    |  xr=x;vr=v;ar=a;transfer=bias;return;
    | end
    | if oldE && ~E
    |  % Transferencia explicita a N1: v_sw en N2 es cero en este mismo cambio.
    |  bias=bias+lastSw;
    | else
    |  bias=bias+min(.25*h,max(-.25*h,-bias));
    | end
    | oldE=E;
    | if mode==4
    |  % El plan AUTO coordinado con izaje aporta su objetivo x/v/a.
    |  goalA=aPlan+1.0*(vPlan-v)+1.0*(xPlan-x);
    | elseif mode==3 || mode==7
    |  goalA=1.0*(manualVelocity-v);
    | elseif mode==9
    |  goalA=1.0*(vPlan-v);
    | else
    |  % READY, transicion a AUTO y parada conservan memoria y frenan a cero.
    |  goalA=-1.0*v;
    | end
    | goalA=min(amax,max(-amax,goalA));
    | aNext=a+min(jmax*h,max(-jmax*h,goalA-a));
    | % Integracion de un segmento de aceleracion lineal (jerk constante).
    | j=(aNext-a)/h;
    | xNext=x+v*h+.5*a*h*h+j*h*h*h/6;
    | vNext=v+.5*(a+aNext)*h;
    | x=xNext;v=vNext;a=aNext;
    | xr=x;vr=v;ar=a;transfer=bias;
    | end
  function [xRef, vxRef, axRef, yRef, vyRef, ayRef] = craneTrajectoryGenerator( ...:
    | function [xRef, vxRef, axRef, yRef, vyRef, ayRef] = craneTrajectoryGenerator( ...
    |     enable, reset, ...
    |     xPos, xVel, xAcc, ...
    |     yPos, yVel, yAcc, ...
    |     xTarget, yTarget, ...
    |     obstacleProfile, ...
    |     suspendedMassKg, loaded, swayAngle, swayRate, Ts)
    | %#codegen
    | % CRANETRAJECTORYGENERATOR
    | % Generador coordinado de referencias de posicion para trolley e izaje.
    | %
    | % Salidas:
    | %   xRef  [m]     : referencia de posicion del trolley.
    | %   vxRef [m/s]   : referencia de velocidad del trolley.
    | %   axRef [m/s^2] : referencia de aceleracion del trolley.
    | %   yRef  [m]     : referencia de posicion del izaje.
    | %   vyRef [m/s]   : referencia de velocidad del izaje.
    | %   ayRef [m/s^2] : referencia de aceleracion del izaje.
    | %
    | % Convencion de coordenadas de la guia:
    | %   x positivo hacia el barco.
    | %   y positivo hacia arriba, con Yt0 = 45 m.
    | %
    | % Uso:
    | %   - Llamar periodicamente con Ts constante.
    | %   - Aplicar reset=true durante al menos una muestra para inicializar.
    | %   - Un flanco ascendente de enable genera una trayectoria nueva.
    | %   - Un cambio de objetivo mientras enable=true provoca replanificacion
    | %     suave desde el estado medido actual.
    | %
    | % Obstaculos:
    | %   obsXMin, obsXMax: intervalo horizontal ocupado por los obstaculos.
    | %   obsYMax: maxima cota superior dentro de ese intervalo.
    | %   Si obsXMax <= obsXMin, se considera que no hay obstaculo intermedio.
    | %
    | % suspendedMassKg es la masa total suspendida:
    | % spreader + headblock + container, entre 15000 y 65000 kg normalmente.
    | 
    | % -------------------------------------------------------------------------
    | % Parametros de la guia y parametros de diseno
    | % -------------------------------------------------------------------------
    | X_MIN = -30.0;
    | X_MAX =  50.0;
    | Y_MIN = -20.0;
    | Y_MAX =  40.0;
    | 
    | VX_MAX = 2.5;       % maxima velocidad de diseno verificable con la planta
    | AX_MAX = 0.3;       % rampa compatible con el seguimiento del accionamiento
    | JX_MAX = 0.5;       % limite de jerk para el traslado productivo
    | 
    | AY_MAX = 0.25;       % conserva tension durante el descenso cargado
    | JY_MAX = 0.10;       % evita transitorios de izaje que aflojen el cable       % Parametro de diseno [m/s^3]
    | % La velocidad cargada se calcula con la masa suspendida.
    | VY_MAX_EMPTY  = 3.00;
    | 
    | YT0 = 45.0;
    | HC = 2.59;
    | WC = 2.44;
    | G = 9.80665;
    | KHWU = 236.0e6;
    | LH0 = 110.0;
    | 
    | VERTICAL_MARGIN = 2.59;       % Parametro de diseno [m]
    | PATH_SWAY_LIMIT = 5.0*pi/180.0;
    | TARGET_CHANGE_TOL = 1.0e-6;
    | MAX_PLAN_TIME = 300.0;  % permite traslados largos a velocidad conservadora
    | 
    | % -------------------------------------------------------------------------
    | % Memoria interna
    | % -------------------------------------------------------------------------
    | persistent initialized prevEnable active validPlan trajectoryTime
    | persistent xCoef xDuration
    | persistent yUpCoef yUpDuration
    | persistent yDownCoef yDownDuration yDownStart
    | persistent savedXTarget savedYTarget
    | 
    | if isempty(initialized)
    |     initialized = true;
    |     prevEnable = false;
    |     active = false;
    |     validPlan = false;
    |     trajectoryTime = 0.0;
    | 
    |     xCoef = zeros(1,6);
    |     xDuration = 0.0;
    |     yUpCoef = zeros(1,6);
    |     yUpDuration = 0.0;
    |     yDownCoef = zeros(1,6);
    |     yDownDuration = 0.0;
    |     yDownStart = 0.0;
    | 
    |     % Inicializacion constante para compatibilidad con MATLAB/PLC Coder.
    |     savedXTarget = 0.0;
    |     savedYTarget = 0.0;
    | end
    | 
    | % Sanitizacion minima de entradas
    | if Ts <= 0.0
    |     TsUse = 0.001;
    | else
    |     TsUse = Ts;
    | end
    | 
    | xGoal = clampValue(xTarget, X_MIN, X_MAX);
    | yGoal = clampValue(yTarget, Y_MIN, Y_MAX);
    | 
    | if reset
    |     prevEnable = false;
    |     active = false;
    |     validPlan = false;
    |     trajectoryTime = 0.0;
    |     savedXTarget = xGoal;
    |     savedYTarget = yGoal;
    |     xRef = clampValue(xPos, X_MIN, X_MAX);
    |     vxRef = clampValue(xVel, -VX_MAX, VX_MAX);
    |     axRef = clampValue(xAcc, -AX_MAX, AX_MAX);
    |     yRef = clampValue(yPos, Y_MIN, Y_MAX);
    |     if loaded
    |         vyLimitReset = hoistSpeedLimit(suspendedMassKg,loaded);
    |     else
    |         vyLimitReset = VY_MAX_EMPTY;
    |     end
    |     vyRef = clampValue(yVel, -vyLimitReset, vyLimitReset);
    |     ayRef = clampValue(yAcc, -AY_MAX, AY_MAX);
    |     return;
    | end
    | 
    | targetChanged = abs(xGoal-savedXTarget) > TARGET_CHANGE_TOL || ...
    |                 abs(yGoal-savedYTarget) > TARGET_CHANGE_TOL;
    | startRequest = enable && (~prevEnable || targetChanged);
    | 
    | if ~enable
    |     active = false;
    |     validPlan = false;
    |     trajectoryTime = 0.0;
    |     prevEnable = false;
    |     xRef = clampValue(xPos, X_MIN, X_MAX);
    |     vxRef = clampValue(xVel, -VX_MAX, VX_MAX);
    |     axRef = clampValue(xAcc, -AX_MAX, AX_MAX);
    |     yRef = clampValue(yPos, Y_MIN, Y_MAX);
    |     if loaded
    |         vyLimitDisabled = hoistSpeedLimit(suspendedMassKg,loaded);
    |     else
    |         vyLimitDisabled = VY_MAX_EMPTY;
    |     end
    |     vyRef = clampValue(yVel, -vyLimitDisabled, vyLimitDisabled);
    |     ayRef = clampValue(yAcc, -AY_MAX, AY_MAX);
    |     return;
    | end
    | 
    | % -------------------------------------------------------------------------
    | % Planificacion en el flanco de enable o ante cambio de objetivo
    | % -------------------------------------------------------------------------
    | if startRequest
    |     savedXTarget = xGoal;
    |     savedYTarget = yGoal;
    |     trajectoryTime = 0.0;
    |     active = true;
    | 
    |     x0 = clampValue(xPos, X_MIN, X_MAX);
    |     y0 = clampValue(yPos, Y_MIN, Y_MAX);
    |     vx0 = clampValue(xVel, -VX_MAX, VX_MAX);
    |     ax0 = clampValue(xAcc, -AX_MAX, AX_MAX);
    |     ay0 = clampValue(yAcc, -AY_MAX, AY_MAX);
    | 
    |     massUse = clampValue(suspendedMassKg, 15000.0, 65000.0);
    |     if loaded
    |         containerHeight = HC;
    |         vyMax = hoistSpeedLimit(suspendedMassKg,loaded);
    |     else
    |         containerHeight = 0.0;
    |         vyMax = VY_MAX_EMPTY;
    |     end
    | 
    |     vy0 = clampValue(yVel, -vyMax, vyMax);
    |     obsXMin=min(x0,xGoal);
    |     obsXMax=max(x0,xGoal);
    |     obsYMax=maximumProfileBetween(obstacleProfile,obsXMin,obsXMax);
    |     hasObstacle=abs(xGoal-x0)>1.0e-6;
    | 
    |     % Altura de izaje necesaria. El estiramiento se obtiene de las
    |     % ecuaciones 4, 5 y 5.a de la guia en equilibrio cuasiestatico.
    |     if hasObstacle
    |         yRequired0 = obsYMax + containerHeight + VERTICAL_MARGIN;
    |         lhEstimate = clampValue(YT0-yRequired0, 5.0, 65.0);
    |         khw = KHWU/(2.0*lhEstimate + LH0);
    |         cableStretch = massUse*G/(4.0*khw);
    |         yRequired = yRequired0 + cableStretch;
    |         yClear = max(max(y0,yGoal),yRequired);
    |         % Se conserva la altura alta de cruce del ciclo original.
    |         yClear = max(yClear,max(obstacleProfile)+5.18);
    |     else
    |         cableStretch = 0.0;
    |         yRequired = max(y0,yGoal);
    |         yClear = yRequired;
    |     end
    | 
    |     % Si el despeje requerido supera el limite mecanico no se inicia.
    |     validPlan = yClear <= Y_MAX + 1.0e-9;
    |     yClear = clampValue(yClear, Y_MIN, Y_MAX);
    | 
    |     % Plan vertical ascendente.
    |     [yUpCoef,yUpDuration,okYUp] = makeMinimumTimeQuintic( ...
    |         y0,vy0,ay0,yClear,0.0,0.0,vyMax,AY_MAX,JY_MAX,TsUse,MAX_PLAN_TIME);
    |     validPlan = validPlan && okYUp;
    | 
    |     % Plan horizontal inicialmente minimo.
    |     [xCoef,xDuration,okX] = makeCruiseProfile( ...
    |         x0,xGoal,VX_MAX,AX_MAX,JX_MAX,MAX_PLAN_TIME);
    |     validPlan = validPlan && okX;
    | 
    |     if validPlan && hasObstacle && xDuration > 0.0
    |         % Se expande horizontalmente la zona por el ancho de la carga y
    |         % por el sway permitido durante la transferencia.
    |         minHoistY = min(min(y0,yGoal),yClear);
    |         maxRopeLength = clampValue(YT0-minHoistY,5.0,65.0);
    |         collisionMargin = 0.5*WC + VERTICAL_MARGIN;
    |         expandedObsMin = obsXMin-collisionMargin;
    |         expandedObsMax = obsXMax+collisionMargin;
    | 
    |         % Si el trolley alcanzaria el obstaculo antes de lograr despeje,
    |         % se aumenta solamente la duracion horizontal. Ambos ejes siguen
    |         % arrancando en t=0, por lo que no hay salto en la referencia.
    |         safe = trajectoryClearsObstacle( ...
    |             xCoef,xDuration,yUpCoef,yUpDuration,yClear, ...
    |             expandedObsMin,expandedObsMax,obstacleProfile, ...
    |             containerHeight,cableStretch,VERTICAL_MARGIN);
    | 
    |         scaleIterations = 0;
    |         while ~safe && xDuration < MAX_PLAN_TIME && scaleIterations < 240
    |             [xCoef,xDuration] = stretchCruiseProfile(xCoef,1.025,MAX_PLAN_TIME);
    | 
    |             safe = trajectoryClearsObstacle( ...
    |                 xCoef,xDuration,yUpCoef,yUpDuration,yClear, ...
    |                 expandedObsMin,expandedObsMax,obstacleProfile, ...
    |                 containerHeight,cableStretch,VERTICAL_MARGIN);
    |             scaleIterations = scaleIterations+1;
    |         end
    | 
    |         validPlan = validPlan && safe;
    | 
    |         % El descenso comienza en cuanto toda la envolvente horizontal de
    |         % la carga ha salido de la zona de obstaculos.
    |         if xGoal >= x0
    |             exitPosition = expandedObsMax;
    |             targetBeyondObstacle = xGoal >= exitPosition;
    |         else
    |             exitPosition = expandedObsMin;
    |             targetBeyondObstacle = xGoal <= exitPosition;
    |         end
    | 
    |         if targetBeyondObstacle
    |             yDownStart = findCrossingTime( ...
    |                 xCoef,xDuration,exitPosition,xGoal>=x0);
    |         else
    |             yDownStart = xDuration;
    |         end
    |     else
    |         yDownStart = xDuration;
    |     end
    | 
    |     % Si no hay obstaculo, se coordina el descenso para terminar junto con
    |     % el trolley, comenzando desde el estado vertical previsto.
    |     if ~hasObstacle
    |         yDownStart = min(xDuration,yUpDuration);
    |     end
    | 
    |     % Estado vertical exacto al comenzar el descenso.
    |     if yDownStart < yUpDuration
    |         [yDown0,vyDown0,ayDown0] = evaluateQuintic( ...
    |             yUpCoef,yDownStart,yUpDuration);
    |     else
    |         yDown0 = yClear;
    |         vyDown0 = 0.0;
    |         ayDown0 = 0.0;
    |     end
    | 
    |     [yDownCoef,yDownDuration,okYDown] = makeMinimumTimeQuintic( ...
    |         yDown0,vyDown0,ayDown0,yGoal,0.0,0.0, ...
    |         vyMax,AY_MAX,JY_MAX,TsUse,MAX_PLAN_TIME);
    |     validPlan = validPlan && okYDown;
    | 
    |     if ~validPlan
    |         active = false;
    |     end
    | end
    | 
    | % -------------------------------------------------------------------------
    | % Evaluacion de la trayectoria
    | % -------------------------------------------------------------------------
    | if active && validPlan
    |     [xRef,vxRef,axRef] = evaluateCruiseProfile( ...
    |         xCoef,trajectoryTime,xDuration);
    | 
    |     if trajectoryTime < yDownStart
    |         [yRef,vyRef,ayRef] = evaluateQuintic( ...
    |             yUpCoef,trajectoryTime,yUpDuration);
    |     else
    |         [yRef,vyRef,ayRef] = evaluateQuintic( ...
    |             yDownCoef,trajectoryTime-yDownStart,yDownDuration);
    |     end
    | 
    |     totalDuration = max(xDuration,yDownStart+yDownDuration);
    |     if trajectoryTime >= totalDuration
    |         xRef = xGoal;
    |         vxRef = 0.0;
    |         axRef = 0.0;
    |         yRef = yGoal;
    |         vyRef = 0.0;
    |         ayRef = 0.0;
    |         % Mantener el plan activo y el reloj saturado para conservar las
    |         % referencias finales hasta reset, disable o replanificacion.
    |         % No volver a las posiciones medidas al terminar la maniobra.
    |         trajectoryTime = totalDuration;
    |     else
    |         finalDescentAtTarget=yDownStart>=xDuration-1.0e-9;
    |         readyForFinalDescent=abs(xPos-xGoal)<=0.08 && abs(xVel)<=0.06 && ...
    |             abs(swayAngle)<=0.0050 && abs(swayRate)<=0.0120;
    |         if finalDescentAtTarget && trajectoryTime>=yDownStart && ~readyForFinalDescent
    |             trajectoryTime=yDownStart;
    |         else
    |             trajectoryTime=trajectoryTime+TsUse;
    |         end
    |     end
    | else
    |     % Comportamiento seguro cuando el plan es inviable: mantener la
    |     % posicion medida y no generar movimiento automatico.
    |     xRef = clampValue(xPos,X_MIN,X_MAX);
    |     vxRef = clampValue(xVel,-VX_MAX,VX_MAX);
    |     axRef = clampValue(xAcc,-AX_MAX,AX_MAX);
    |     yRef = clampValue(yPos,Y_MIN,Y_MAX);
    |     if loaded
    |         vyLimitInvalid = hoistSpeedLimit(suspendedMassKg,loaded);
    |     else
    |         vyLimitInvalid = VY_MAX_EMPTY;
    |     end
    |     vyRef = clampValue(yVel,-vyLimitInvalid,vyLimitInvalid);
    |     ayRef = clampValue(yAcc,-AY_MAX,AY_MAX);
    | end
    | 
    | xRef = clampValue(xRef,X_MIN,X_MAX);
    | vxRef = clampValue(vxRef,-VX_MAX,VX_MAX);
    | axRef = clampValue(axRef,-AX_MAX,AX_MAX);
    | yRef = clampValue(yRef,Y_MIN,Y_MAX);
    | if loaded
    |     vyLimitOutput = hoistSpeedLimit(suspendedMassKg,loaded);
    | else
    |     vyLimitOutput = VY_MAX_EMPTY;
    | end
    | vyRef = clampValue(vyRef,-vyLimitOutput,vyLimitOutput);
    | ayRef = clampValue(ayRef,-AY_MAX,AY_MAX);
    | prevEnable = enable;
    | end
    | 
    | % =========================================================================
    | % Funciones auxiliares compatibles con generacion de codigo
    | % =========================================================================
    | 
    | function maximumY = maximumProfileBetween(profile,xStart,xEnd)
    | xMin=-30.0; slotWidth=2.44; halfWidth=1.22;
    | pathMin=min(xStart,xEnd)-halfWidth;
    | pathMax=max(xStart,xEnd)+halfWidth;
    | maximumY=-20.0;
    | for k=1:33
    |     slotX=xMin+double(k-1)*slotWidth;
    |     if slotX+halfWidth>=pathMin && slotX-halfWidth<=pathMax
    |         maximumY=max(maximumY,profile(k));
    |     end
    | end
    | end
    | 
    | function value = clampValue(value,lowerLimit,upperLimit)
    | value = min(upperLimit,max(lowerLimit,value));
    | end
    | 
    | function [profile,duration,ok] = makeCruiseProfile( ...
    |     xStart,xGoal,vMax,aMax,jMax,maxTime)
    | distance=abs(xGoal-xStart);
    | if distance<1.0e-10
    |     profile=[xGoal,xGoal,0.0,0.0,0.0,0.0];
    |     duration=0.0; ok=true; return;
    | end
    | direction=sign(xGoal-xStart);
    | rampA=pi*vMax/(2.0*max(aMax,1.0e-6));
    | rampJ=pi*sqrt(vMax/(2.0*max(jMax,1.0e-6)));
    | rampDuration=max(0.25,max(rampA,rampJ));
    | if distance>=vMax*rampDuration
    |     cruiseVelocity=vMax;
    |     cruiseDuration=distance/cruiseVelocity-rampDuration;
    | else
    |     cruiseVelocity=distance/rampDuration;
    |     cruiseDuration=0.0;
    | end
    | duration=2.0*rampDuration+cruiseDuration;
    | profile=[xStart,xGoal,direction,cruiseVelocity,rampDuration,cruiseDuration];
    | ok=duration<=maxTime;
    | end
    | 
    | function [profile,duration] = stretchCruiseProfile(profile,scale,maxTime)
    | oldDuration=2.0*profile(5)+profile(6);
    | newDuration=min(maxTime,scale*oldDuration);
    | actualScale=max(1.0,newDuration/max(oldDuration,1.0e-9));
    | profile(4)=profile(4)/actualScale;
    | profile(5)=profile(5)*actualScale;
    | profile(6)=profile(6)*actualScale;
    | duration=2.0*profile(5)+profile(6);
    | end
    | 
    | function [position,velocity,acceleration] = evaluateCruiseProfile(profile,time,duration)
    | xStart=profile(1); xGoal=profile(2); direction=profile(3);
    | vCruise=profile(4); rampDuration=profile(5);
    | cruiseDuration=profile(6);
    | if duration<=0.0 || direction==0.0
    |     position=xGoal; velocity=0.0; acceleration=0.0; return;
    | end
    | t=min(duration,max(0.0,time));
    | if t<rampDuration
    |     angle=pi*t/rampDuration;
    |     travelled=0.5*vCruise*(t-rampDuration*sin(angle)/pi);
    |     speed=0.5*vCruise*(1.0-cos(angle));
    |     accel=0.5*vCruise*pi*sin(angle)/rampDuration;
    | elseif t<rampDuration+cruiseDuration
    |     travelled=0.5*vCruise*rampDuration+vCruise*(t-rampDuration);
    |     speed=vCruise; accel=0.0;
    | elseif t<duration
    |     tau=t-rampDuration-cruiseDuration;
    |     angle=pi*tau/rampDuration;
    |     travelled=0.5*vCruise*rampDuration+vCruise*cruiseDuration+...
    |         0.5*vCruise*(tau+rampDuration*sin(angle)/pi);
    |     speed=0.5*vCruise*(1.0+cos(angle));
    |     accel=-0.5*vCruise*pi*sin(angle)/rampDuration;
    | else
    |     position=xGoal; velocity=0.0; acceleration=0.0; return;
    | end
    | position=xStart+direction*travelled;
    | velocity=direction*speed; acceleration=direction*accel;
    | end
    | 
    | function [coef,duration,ok] = makeMinimumTimeQuintic( ...
    |     p0,v0,a0,pf,vf,af,vMax,aMax,jMax,Ts,maxTime)
    | 
    | if abs(pf-p0) < 1.0e-10 && abs(v0-vf) < 1.0e-8 && ...
    |         abs(a0-af) < 1.0e-7
    |     coef = [pf,0.0,0.0,0.0,0.0,0.0];
    |     duration = 0.0;
    |     ok = true;
    |     return;
    | end
    | 
    | durationHigh = max(10.0*Ts,0.05);
    | coef = quinticCoefficients(p0,v0,a0,pf,vf,af,durationHigh);
    | 
    | while ~profileWithinLimits(coef,durationHigh,vMax,aMax,jMax) && ...
    |         durationHigh < maxTime
    |     durationHigh = min(maxTime,2.0*durationHigh);
    |     coef = quinticCoefficients(p0,v0,a0,pf,vf,af,durationHigh);
    | end
    | 
    | ok = profileWithinLimits(coef,durationHigh,vMax,aMax,jMax);
    | if ~ok
    |     duration = durationHigh;
    |     return;
    | end
    | 
    | durationLow = max(Ts,0.001);
    | for iteration = 1:48
    |     durationMid = 0.5*(durationLow+durationHigh);
    |     coefMid = quinticCoefficients(p0,v0,a0,pf,vf,af,durationMid);
    |     if profileWithinLimits(coefMid,durationMid,vMax,aMax,jMax)
    |         durationHigh = durationMid;
    |         coef = coefMid;
    |     else
    |         durationLow = durationMid;
    |     end
    | end
    | 
    | duration = durationHigh;
    | end
    | 
    | function coef = quinticCoefficients(p0,v0,a0,pf,vf,af,T)
    | if T <= 0.0
    |     coef = [pf,0.0,0.0,0.0,0.0,0.0];
    |     return;
    | end
    | 
    | T2 = T*T;
    | T3 = T2*T;
    | T4 = T3*T;
    | T5 = T4*T;
    | 
    | c0 = p0;
    | c1 = v0;
    | c2 = 0.5*a0;
    | c3 = (20.0*(pf-p0) - (8.0*vf+12.0*v0)*T ...
    |       - (3.0*a0-af)*T2)/(2.0*T3);
    | c4 = (30.0*(p0-pf) + (14.0*vf+16.0*v0)*T ...
    |       + (3.0*a0-2.0*af)*T2)/(2.0*T4);
    | c5 = (12.0*(pf-p0) - (6.0*vf+6.0*v0)*T ...
    |       - (a0-af)*T2)/(2.0*T5);
    | 
    | coef = [c0,c1,c2,c3,c4,c5];
    | end
    | 
    | function [position,velocity,acceleration] = evaluateQuintic(coef,time,duration)
    | if duration <= 0.0
    |     position = coef(1);
    |     velocity = 0.0;
    |     acceleration = 0.0;
    |     return;
    | end
    | 
    | t = clampValue(time,0.0,duration);
    | c0 = coef(1);
    | c1 = coef(2);
    | c2 = coef(3);
    | c3 = coef(4);
    | c4 = coef(5);
    | c5 = coef(6);
    | 
    | position = c0+t*(c1+t*(c2+t*(c3+t*(c4+t*c5))));
    | velocity = c1+t*(2.0*c2+t*(3.0*c3+t*(4.0*c4+t*5.0*c5)));
    | acceleration = 2.0*c2+t*(6.0*c3+t*(12.0*c4+t*20.0*c5));
    | end
    | 
    | function jerk = evaluateJerk(coef,time,duration)
    | if duration <= 0.0
    |     jerk = 0.0;
    |     return;
    | end
    | t = clampValue(time,0.0,duration);
    | jerk = 6.0*coef(4)+t*(24.0*coef(5)+t*60.0*coef(6));
    | end
    | 
    | function ok = profileWithinLimits(coef,duration,vMax,aMax,jMax)
    | if duration <= 0.0
    |     ok = true;
    |     return;
    | end
    | 
    | ok = true;
    | for sample = 0:240
    |     t = duration*double(sample)/240.0;
    |     [~,velocity,acceleration] = evaluateQuintic(coef,t,duration);
    |     jerk = evaluateJerk(coef,t,duration);
    |     if abs(velocity) > vMax*(1.0+1.0e-8) || ...
    |        abs(acceleration) > aMax*(1.0+1.0e-8) || ...
    |        abs(jerk) > jMax*(1.0+1.0e-8)
    |         ok = false;
    |         return;
    |     end
    | end
    | end
    | 
    | function safe = trajectoryClearsObstacle( ...
    |     xCoef,xDuration,yCoef,yDuration,yHold, ...
    |     obstacleMin,obstacleMax,obstacleProfile, ...
    |     containerHeight,cableStretch,verticalMargin)
    | 
    | safe = true;
    | for sample = 0:400
    |     t = xDuration*double(sample)/400.0;
    |     [x,~,~] = evaluateCruiseProfile(xCoef,t,xDuration);
    | 
    |     if x >= obstacleMin && x <= obstacleMax && abs(x-xCoef(1))>0.02 && abs(x-xCoef(1))>0.02 && abs(x-xCoef(1))>0.02 && abs(x-xCoef(1))>0.02 && abs(x-xCoef(1))>0.02 && abs(x-xCoef(1))>0.02 && abs(x-xCoef(1))>0.02
    |         if t < yDuration
    |             [y,~,~] = evaluateQuintic(yCoef,t,yDuration);
    |         else
    |             y = yHold;
    |         end
    | 
    |         obstacleHeight=maximumProfileBetween(obstacleProfile,x,x);
    |         bottomHeight = y-cableStretch-containerHeight;
    |         if bottomHeight < obstacleHeight+verticalMargin-1.0e-8
    |             safe = false;
    |             return;
    |         end
    |     end
    | end
    | end
    | 
    | function crossingTime = findCrossingTime(coef,duration,position,positiveDirection)
    | crossingTime = duration;
    | if duration <= 0.0
    |     return;
    | end
    | 
    | previousTime = 0.0;
    | [previousPosition,~,~] = evaluateCruiseProfile(coef,0.0,duration);
    | 
    | for sample = 1:400
    |     currentTime = duration*double(sample)/400.0;
    |     [currentPosition,~,~] = evaluateCruiseProfile( ...
    |         coef,currentTime,duration);
    | 
    |     if positiveDirection
    |         crossed = previousPosition < position && currentPosition >= position;
    |     else
    |         crossed = previousPosition > position && currentPosition <= position;
    |     end
    | 
    |     if crossed
    |         low = previousTime;
    |         high = currentTime;
    |         for iteration = 1:32
    |             middle = 0.5*(low+high);
    |             [middlePosition,~,~] = evaluateCruiseProfile(coef,middle,duration);
    |             if positiveDirection
    |                 if middlePosition >= position
    |                     high = middle;
    |                 else
    |                     low = middle;
    |                 end
    |             else
    |                 if middlePosition <= position
    |                     high = middle;
    |                 else
    |                     low = middle;
    |                 end
    |             end
    |         end
    |         crossingTime = high;
    |         return;
    |     end
    | 
    |     previousTime = currentTime;
    |     previousPosition = currentPosition;
    | end
    | end
    | 
    | 
    | function vMax = hoistSpeedLimit(totalMassKg,loaded)
    | if loaded
    |     massUse=clampValue(totalMassKg,15000.0,65000.0);
    |     vMax=min(3.0,max(1.5,97500.0/massUse));
    | else
    |     vMax=3.0;
    | end
    | end
  function [xRef,vxRef,axRef,yRef,vyRef,ayRef] = referenciasManual(x,vx,y,vy,vxCmd,vyCmd,Ts):
    | function [xRef,vxRef,axRef,yRef,vyRef,ayRef] = referenciasManual(x,vx,y,vy,vxCmd,vyCmd,Ts)
    | %#codegen
    | persistent previousVxRef previousVyRef
    | if isempty(previousVxRef)
    |     previousVxRef=0.0; previousVyRef=0.0;
    | end
    | TsUse=max(0.001,Ts);
    | vxTarget=min(4.0,max(-4.0,vxCmd));
    | vyTarget=min(3.0,max(-3.0,vyCmd));
    | deltaVx=min(0.8*TsUse,max(-0.8*TsUse,vxTarget-previousVxRef));
    | deltaVy=min(0.75*TsUse,max(-0.75*TsUse,vyTarget-previousVyRef));
    | vxRef=min(4.0,max(-4.0,previousVxRef+deltaVx));
    | vyRef=min(3.0,max(-3.0,previousVyRef+deltaVy));
    | axRef=min(0.8,max(-0.8,deltaVx/TsUse));
    | ayRef=min(0.75,max(-0.75,deltaVy/TsUse));
    | xRef=min(50.0,max(-30.0,x+vxRef*TsUse));
    | yRef=min(40.0,max(-20.0,y+vyRef*TsUse));
    | previousVxRef=vxRef; previousVyRef=vyRef;
    | end
  function [xRef,vxRef,axRef,yRef,vyRef,ayRef] = referenciasBumpless(x,vx,y,vy,vxTarget,vyTarget,Ts):
    | function [xRef,vxRef,axRef,yRef,vyRef,ayRef] = referenciasBumpless(x,vx,y,vy,vxTarget,vyTarget,Ts)
    | %#codegen
    | TsUse=max(0.001,Ts);
    | dvx=min(0.8*TsUse,max(-0.8*TsUse,vxTarget-vx));
    | dvy=min(0.75*TsUse,max(-0.75*TsUse,vyTarget-vy));
    | vxRef=min(4.0,max(-4.0,vx+dvx));
    | vyRef=min(3.0,max(-3.0,vy+dvy));
    | axRef=dvx/TsUse; ayRef=dvy/TsUse;
    | xRef=min(50.0,max(-30.0,x+vxRef*TsUse));
    | yRef=min(40.0,max(-20.0,y+vyRef*TsUse));
    | end
  function [xRef,vxRef,axRef,yRef,vyRef,ayRef]=referenciaDescensoFinal(xTarget,y,vy,vyCmd,Ts):
    | function [xRef,vxRef,axRef,yRef,vyRef,ayRef]=referenciaDescensoFinal(xTarget,y,vy,vyCmd,Ts)
    | %#codegen
    | persistent previousVyRef
    | if isempty(previousVyRef), previousVyRef=0.0; end
    | TsUse=max(0.001,Ts);
    | xRef=min(50.0,max(-30.0,xTarget));
    | vxRef=0.0; axRef=0.0;
    | vyTarget=min(3.0,max(-3.0,vyCmd));
    | deltaVy=min(0.05*TsUse,max(-0.05*TsUse,vyTarget-previousVyRef));
    | vyRef=min(3.0,max(-3.0,previousVyRef+deltaVy));
    | ayRef=min(0.05,max(-0.05,deltaVy/TsUse));
    | yRef=min(40.0,max(-20.0,y+vyRef*TsUse));
    | previousVyRef=vyRef;
    | end
  function masa = Estimar_Masa(F_hw, TLK_Close_FB):
    | function masa = Estimar_Masa(F_hw, TLK_Close_FB)
    | 
    |     G = 9.80665;
    |     MS = 15000;
    |     
    |     if TLK_Close_FB
    |         masa_total = 2*F_hw / G;
    |         masa = max(0, masa_total - MS);
    |     else
    |         masa = 0;
    |     end
    | end
